simulink model "lab3_1"  (R2021b)
settings: Solver=VariableStepAuto  StartTime=0.0  StopTime=30.0  RelTol=10e-10  AbsTol=10e-10
values from neighbouring files (symbols this model uses):
  dbar = g*sin(thetta)    [lab3.m]
  vdes = 14    [lab3.m]
libraries: cstblocks x2
settings Model: Creator=jiayizhou  LastModifiedBy=jiayizhou

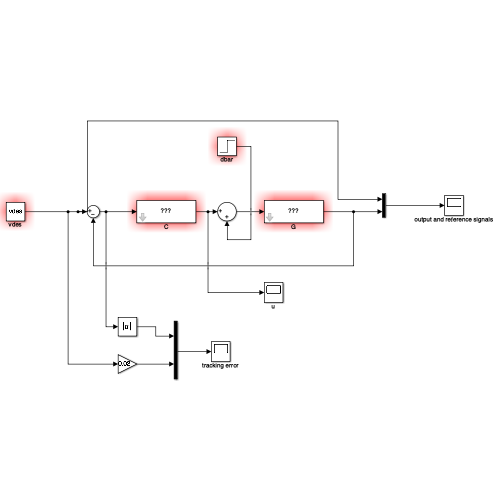
[thumbnail: Simulink's stored preview of the top-level diagram]
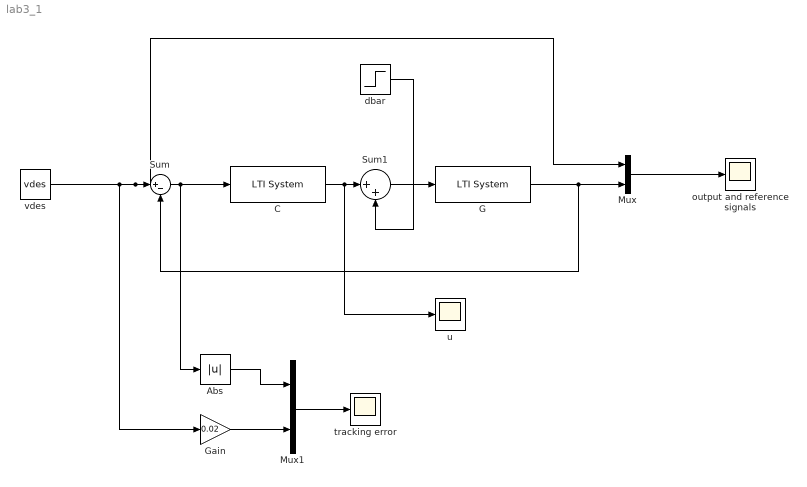
== system lab3_1 ==
  Abs : Abs
  C : cstblocks/LTI System  sys=C  IC=[]
  G : cstblocks/LTI System  sys=G  IC=[]
  Gain : Gain  Gain=0.02
  Mux : Mux  Inputs=2
  Mux1 : Mux  Inputs=2
  Sum : Sum  Inputs=|+-
  Sum1 : Sum  Inputs=|++
  dbar : Step  Time=15  After=dbar  SampleTime=0
  output and reference signals : Scope
  tracking error : Scope
  u : Scope
  vdes : Constant  Value=vdes
  wires:
  vdes/1 -> Gain/1, Mux/1, Sum/1
  Sum/1 -> Abs/1, C/1
  C/1 -> u/1, Sum1/1
  Sum1/1 -> G/1
  dbar/1 -> Sum1/2
  G/1 -> Mux/2, Sum/2
  Mux/1 -> output and reference signals/1
  Abs/1 -> Mux1/1
  Gain/1 -> Mux1/2
  Mux1/1 -> tracking error/1
